simulink model "EarlyReturn12"  (R2020b)
settings: Solver=VariableStepAuto  StartTime=0.0  StopTime=0.1  RelTol=1e-3
settings Model: Creator=BEAR  LastModifiedBy=apple
settings DataIOCC: ReturnWorkspaceOutputs=off
settings DebuggingCC: ArithmeticOperatorsInVariantConditions=warning
settings SFSimCC: SimUseLocalCustomCode=off  CustomCodeUndefinedFunction=UseInterfaceOnly
settings RTWCC: RTWUseLocalCustomCode=off

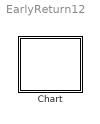
== system EarlyReturn12 ==
  Chart : Stateflow chart  TreatAsAtomicUnit=on

== stateflow chart EarlyReturn12/Chart ==
  state A
    en: E;fprintf("enA_done")
  state B
    en: fprintf("enB")
  state C
    en: fprintf("enC")
  (default) -> A
  A -> B : E
  B -> C
  events: E local FUNCTION_CALL_EVENT
